simulink model "HQEV_MiL_20160830_integrate"  (Simulink 8.3)
settings: Solver=FixedStepDiscrete  StartTime=0.0  StopTime=inf  FixedStep=0.01  RelTol=1e-3
PostLoadFcn:
  | , if any(exist('dsrtsu_mdlpostloadfcn', 'file') == [2, 3, 6]), try dsrtsu_mdlpostloadfcn('Execute', bdroot); catch fprintf('Error in PostLoadFcn (dsrtsu_mdlpostloadfcn) for model "%s":\n %s\n', bdroot, lasterr); end, end,
values from neighbouring files (symbols this model uses):
  Bat_C_Ah = 36    [parameter_V1.mat]
  Bat_ocv_xIndex = [5 10 20 30 40 50 60 70 80 90 95]    [parameter_V1.mat]
  Bat_ocv_z = [329 332 340 345 347 351 358 372 377 386 391]    [parameter_V1.mat]
  Bat_R_ohm_z = [4.41 3.46 1.57 1.07 0.76 0.63 0.55 0.44 0.41 0.4 0.4 3.14 ... (66 elements, 11x6)]    [parameter_V1.mat]
  Bat_SOC_Init = 90    [parameter_V1.mat]
  Env_hum_pct_Ambient = 30    [parameter_V1.mat]
  Env_Slope_deg = 0    [parameter_V1.mat]
  Env_Temp_degC_Ambient = 25    [parameter_V1.mat]
  Env_v_kmph_HWind = 0    [parameter_V1.mat]
  Reducer_F_i = 7.23    [parameter_V1.mat]
  Reducer_R_i = 7.23    [parameter_V1.mat]
  Veh =     [parameter_V1.mat]
  Veh_A_m2_Fr = 2.246    [parameter_V1.mat]
  Veh_F_Brake =     [parameter_V1.mat]
  Veh_fac_AirDrag = 0.326    [parameter_V1.mat]
  Veh_fac_WhDragFrict_0 = 0.011    [parameter_V1.mat]
  Veh_g_mps2_C = 9.81    [parameter_V1.mat]
  Veh_GainBrake =     [parameter_V1.mat]
  Veh_h_m_COGHigh = 0.5    [parameter_V1.mat]
  Veh_J_kgm2_Wh = 1.3635    [parameter_V1.mat]
  Veh_L_m_AxlBas = 2.63    [parameter_V1.mat]
  Veh_M_kg = 1427    [parameter_V1.mat]
  Veh_mu_Brake = 0.4    [parameter_V1.mat]
  Veh_mu_Tyre =     [parameter_V1.mat]
  Veh_num_FrictPair = 8    [parameter_V1.mat]
  Veh_pct_Brk = 70    [parameter_V1.mat]
  Veh_r_dyn =     [parameter_V1.mat]
  Veh_r_m_BrkDisk = 0.136    [parameter_V1.mat]
  Veh_rho_kgpm3_Air = 1.2258    [parameter_V1.mat]
undefined symbols (not defined in the file or in its folder): DiscIntNeverNeededParam, p_bool_False_M, p_bool_True_M
libraries: BaseOperationLib_Browser x38, simulink x9, DTQC_lib x1, ERR_lib x1, MQM_lib x1, PTCL_lib x1, PUD_lib x1, TQD_lib x1, TQR_lib x1, VMM_lib x1, ACCA_lib x1, BBCA_lib x1
(part 4 of 15)

== system HQEV_MiL_20160830_integrate/MiL/Test_Integration/IC/IC ==
  In1 : Inport
  Bus Creator : BusCreator  Inputs=2
  Subsystem : Subsystem
  IC : Outport
  wires:
  In1/1 -> Subsystem/1(In1)
  Subsystem/1(HandBrakeSt) -> Bus Creator/1  "HandBrakeSt"
  Subsystem/2(DDSPS) -> Bus Creator/2  "DDSPS"
  Bus Creator/1 -> IC/1

== system HQEV_MiL_20160830_integrate/MiL/Test_Integration/MCU_FF/MCU ==
  In1 : Inport
  Bus Creator : BusCreator  Inputs=2
  MCU : Subsystem
  Signal : Subsystem
  Out1 : Outport
  wires:
  In1/1 -> Bus Creator/1, MCU/1(In1)
  MCU/1(out) -> Bus Creator/2
  Bus Creator/1 -> Signal/1(bus)
  Signal/1(Out1) -> Out1/1

== system HQEV_MiL_20160830_integrate/MiL/Test_Integration/MCU_RR/MCU ==
  In1 : Inport
  Bus Creator : BusCreator  Inputs=2
  MCU : Subsystem
  Signal : Subsystem
  Out1 : Outport
  wires:
  In1/1 -> Bus Creator/1, MCU/1(In1)
  MCU/1(Out1) -> Bus Creator/2
  Signal/1(Out1) -> Out1/1
  Bus Creator/1 -> Signal/1(in)

== system HQEV_MiL_20160830_integrate/MiL/Test_Integration/Motor_FF/Motor ==
  In1 : Inport
  Bus Creator : BusCreator  Inputs=6
  Bus Selector : BusSelector  OutputSignals=Reducer_F.FD1_spd_in,MCU_F.MCU1_trq_req,HCU.HCU_RapidDischargeCmdToMCU1,Battery.Battery_Voltage,BMS.BMS_MainPlusContactorCoilState,BMS.BMS_PrechargeContactorCoilState,BMS.BMS_MainMinusContactorCoilState,BMS.BMS_ChargePlusContactorCoilState,BMS.BMS_ChargeMinusContactorCoilState,Charger.Charger_Status
  Motor : Subsystem
  Out1 : Outport
  wires:
  In1/1 -> Bus Selector/1
  Motor/1(n_Motor) -> Bus Creator/1  "EM1_spd"
  Motor/2(P_Motor_elec) -> Bus Creator/2  "EM1_pwr_elec"
  Motor/3(T_out) -> Bus Creator/3  "EM1_trq_out"
  Motor/4(J_out) -> Bus Creator/4  "EM1_J_out"
  Motor/5(P_Motor_loss) -> Bus Creator/5  "EM1_pwr_loss"
  Motor/6(U_TMCap) -> Bus Creator/6  "EM1_U"
  Bus Creator/1 -> Out1/1
  Bus Selector/1 -> Motor/1(n_FD_in)  "<FD1_spd_in>"
  Bus Selector/2 -> Motor/2(T_req)  "<MCU1_trq_req>"
  Bus Selector/5 -> Motor/5(MainPos_Contactor)  "<BMS_MainPlusContactorCoilState>"
  Bus Selector/6 -> Motor/6(PreCharg_Contactor)  "<BMS_PrechargeContactorCoilState>"
  Bus Selector/7 -> Motor/7(MainNeg_Contactor)  "<BMS_MainMinusContactorCoilState>"
  Bus Selector/3 -> Motor/3(RapidDischargeEnable)  "<HCU_RapidDischargeCmdToMCU1>"
  Bus Selector/4 -> Motor/4(Battery_Voltage)  "<Battery_Voltage>"
  Bus Selector/8 -> Motor/8(BMS_ChargePlusContactorCoilState)  "<BMS_ChargePlusContactorCoilState>"
  Bus Selector/9 -> Motor/9(BMS_ChargeMinusContactorCoilState)  "<BMS_ChargeMinusContactorCoilState>"
  Bus Selector/10 -> Motor/10(Charger_Status)  "<Charger_Status>"

== system HQEV_MiL_20160830_integrate/MiL/Test_Integration/Motor_RR/Motor ==
  In1 : Inport
  Bus Creator : BusCreator  Inputs=6
  Bus Selector : BusSelector  OutputSignals=Reducer_R.FD2_spd_in,MCU_R.MCU2_trq_req,HCU.HCU_RapidDischargeCmdToMCU2,Battery.Battery_Voltage,BMS.BMS_MainPlusContactorCoilState,BMS.BMS_PrechargeContactorCoilState,BMS.BMS_MainMinusContactorCoilState,BMS.BMS_ChargePlusContactorCoilState,BMS.BMS_ChargeMinusContactorCoilState,Charger.Charger_Status
  Motor1 : Subsystem
  Out1 : Outport
  wires:
  In1/1 -> Bus Selector/1
  Motor1/1(n_Motor) -> Bus Creator/1  "EM2_spd"
  Motor1/2(P_Motor_elec) -> Bus Creator/2  "EM2_pwr_elec"
  Motor1/3(T_out) -> Bus Creator/3  "EM2_trq_out"
  Motor1/4(J_out) -> Bus Creator/4  "EM2_J_out"
  Motor1/5(P_Motor_loss) -> Bus Creator/5  "EM2_pwr_loss"
  Motor1/6(U_TMCap) -> Bus Creator/6  "EM2_U"
  Bus Creator/1 -> Out1/1
  Bus Selector/1 -> Motor1/1(n_FD_in)  "<FD2_spd_in>"
  Bus Selector/2 -> Motor1/2(T_req)  "<MCU2_trq_req>"
  Bus Selector/3 -> Motor1/3(RapidDischargeEnable)  "<HCU_RapidDischargeCmdToMCU2>"
  Bus Selector/4 -> Motor1/4(Battery_Voltage)  "<Battery_Voltage>"
  Bus Selector/5 -> Motor1/5(MainPos_Contactor)  "<BMS_MainPlusContactorCoilState>"
  Bus Selector/6 -> Motor1/6(PreCharg_Contactor)  "<BMS_PrechargeContactorCoilState>"
  Bus Selector/7 -> Motor1/7(MainNeg_Contactor)  "<BMS_MainMinusContactorCoilState>"
  Bus Selector/8 -> Motor1/8(BMS_ChargePlusContactorCoilState)  "<BMS_ChargePlusContactorCoilState>"
  Bus Selector/9 -> Motor1/9(BMS_ChargeMinusContactorCoilState)  "<BMS_ChargeMinusContactorCoilState>"
  Bus Selector/10 -> Motor1/10(Charger_Status)  "<Charger_Status>"

== system HQEV_MiL_20160830_integrate/MiL/Test_Integration/Reducer_F/FinalDrive ==
  In1 : Inport
  Bus Creator : BusCreator  Inputs=3
  Bus Selector1 : BusSelector  OutputSignals=Motor_F.EM1_trq_out,Vehicle.n_Wh,Motor_F.EM1_J_out
  FinalDrive : Subsystem
  Out : Outport
  wires:
  FinalDrive/1("T_out ") -> Bus Creator/1  "FD1_trq_out"
  FinalDrive/2(n_in) -> Bus Creator/2  "FD1_spd_in"
  FinalDrive/3("J_out ") -> Bus Creator/3  "FD1_J_out"
  Bus Creator/1 -> Out/1
  In1/1 -> Bus Selector1/1
  Bus Selector1/1 -> FinalDrive/1(T_in)  "<EM1_trq_out>"
  Bus Selector1/2 -> FinalDrive/2(n_Wheel)  "<n_Wh>"
  Bus Selector1/3 -> FinalDrive/3(J_in)  "<EM1_J_out>"

== system HQEV_MiL_20160830_integrate/MiL/Test_Integration/Reducer_R/FinalDrive ==
  In1 : Inport
  Bus Creator : BusCreator  Inputs=3
  Bus Selector1 : BusSelector  OutputSignals=Motor_R.EM2_trq_out,Vehicle.n_Wh,Motor_R.EM2_J_out
  FinalDrive : Subsystem
  Out : Outport
  wires:
  Bus Selector1/3 -> FinalDrive/3(J_in [kg*m^2])  "<EM2_J_out>"
  Bus Selector1/2 -> FinalDrive/2(n_Wheel)  "<n_Wh>"
  Bus Selector1/1 -> FinalDrive/1(T_in)  "<EM2_trq_out>"
  In1/1 -> Bus Selector1/1
  Bus Creator/1 -> Out/1
  FinalDrive/3(J_out [kg*m^2]) -> Bus Creator/3  "FD2_J_out"
  FinalDrive/2(n_in) -> Bus Creator/2  "FD2_spd_in"
  FinalDrive/1(T_out [Nm]) -> Bus Creator/1  "FD2_trq_out"

== system HQEV_MiL_20160830_integrate/MiL/Test_Integration/Thermal/Thermal ==
  In1 : Inport
  Bus Creator : BusCreator  Inputs=5
  Bus Selector : BusSelector  OutputSignals=HCU.EM1PumpCmd_pct,HCU.EM2PumpCmd_pct,Motor_F.EM1_pwr_loss,Motor_R.EM2_pwr_loss,HCU.LowSpdFanCmd_na,HCU.HighSpdFanCmd_na,Charger.Charger_pwr_out,DCDC.DCDC_pwr_Loss,HCU.BatPumpCmd_pct,HCU.HCU_BatteryPackCoolRequest,HCU.PTC_PWM_pct,Battery.Battery_Power_loss,IO.BatTempIndex
  Subsystem : Subsystem
  Out1 : Outport
  wires:
  Bus Creator/1 -> Out1/1
  Subsystem/1(Motor_F_Temp) -> Bus Creator/1  "Motor_F_Temp"
  Subsystem/2(Motor_R_Temp) -> Bus Creator/2  "Motor_R_Temp"
  Subsystem/3(DCDC_Temp) -> Bus Creator/3  "DCDC_Temp"
  Subsystem/4(Charger_Temp) -> Bus Creator/4  "Charger_Temp"
  Subsystem/5(Battery_Temp) -> Bus Creator/5  "Battery_Temp"
  In1/1 -> Bus Selector/1
  Bus Selector/1 -> Subsystem/1(PWM_Pump1)  "<EM1PumpCmd_pct>"
  Bus Selector/2 -> Subsystem/2(PWM_Pump2)  "<EM2PumpCmd_pct>"
  Bus Selector/3 -> Subsystem/3(pwr_Motor1Loss)  "<EM1_pwr_loss>"
  Bus Selector/4 -> Subsystem/4(pwr_Motor2Loss)  "<EM2_pwr_loss>"
  Bus Selector/5 -> Subsystem/5(LowSpdFan_na)  "<LowSpdFanCmd_na>"
  Bus Selector/6 -> Subsystem/6(HighSpdFan_na)  "<HighSpdFanCmd_na>"
  Bus Selector/7 -> Subsystem/7(pwr_ChargerLoss)  "<Charger_pwr_out>"
  Bus Selector/8 -> Subsystem/8(pwr_DCDCLoss)  "<DCDC_pwr_Loss>"
  Bus Selector/9 -> Subsystem/9(PWM_BatteryPump)  "<BatPumpCmd_pct>"
  Bus Selector/10 -> Subsystem/10(AC_OnOff)  "<HCU_BatteryPackCoolRequest>"
  Bus Selector/11 -> Subsystem/11(PWM_PTC)  "<PTC_PWM_pct>"
  Bus Selector/12 -> Subsystem/12(pwr_BatteryLoss)  "<Battery_Power_loss>"
  Bus Selector/13 -> Subsystem/13(BatTempIndex)  "<BatTempIndex>"

== system HQEV_MiL_20160830_integrate/MiL/Test_Integration/Vehicle/Vehicle ==
  In1 : Inport
  Add : Sum
  Bus Creator : BusCreator
  Bus Selector : BusSelector  OutputSignals=Reducer_F.FD1_trq_out,Reducer_R.FD2_trq_out,Drv.signal1.BrkPed_pct,Env.v_Hwind,Reducer_F.FD1_J_out,Reducer_R.FD2_J_out
  Constant1 : Constant  Value=0
  Constant3 : Constant  Value=0
  Vehicle : Subsystem
  Out2 : Outport
  wires:
  Vehicle/1(n_Wh) -> Bus Creator/1  "n_Wh"
  Vehicle/2(dist [km]) -> Bus Creator/2  "dist"
  Vehicle/3(v_Veh [km/h]) -> Bus Creator/3  "v_Veh"
  Constant3/1 -> Vehicle/6(m_add)
  Bus Creator/1 -> Out2/1  "Vehicle"
  Vehicle/4(acc) -> Bus Creator/4  "acc"
  In1/1 -> Bus Selector/1
  Bus Selector/1 -> Vehicle/1("T_inFront ")  "<FD1_trq_out>"
  Bus Selector/2 -> Vehicle/2("T_inRear ")  "<FD2_trq_out>"
  Bus Selector/3 -> Vehicle/3(Sig_Brake)  "<BrkPed_pct>"
  Bus Selector/4 -> Vehicle/4(v_Hwind_mps)  "<v_Hwind>"
  Bus Selector/5 -> Add/1  "<FD1_J_out>"
  Bus Selector/6 -> Add/2  "<FD2_J_out>"
  Add/1 -> Vehicle/5(J_in)
  Constant1/1 -> Vehicle/7(Slope_deg)

== system HQEV_MiL_20160830_integrate/MiL/Test_Integration/AC/AirConditioning/ACIndication ==
  Constant8 : Constant  Value=0
  out : Outport
  wires:
  Constant8/1 -> out/1

== system HQEV_MiL_20160830_integrate/MiL/Test_Integration/AC/AirConditioning/AC_CompressorOnRequest ==
  Constant : Constant  Value=0
  out : Outport
  wires:
  Constant/1 -> out/1

== system HQEV_MiL_20160830_integrate/MiL/Test_Integration/AC/AirConditioning/AC_FanRequest ==
  Constant6 : Constant  Value=0
  out : Outport
  wires:
  Constant6/1 -> out/1

== system HQEV_MiL_20160830_integrate/MiL/Test_Integration/AC/AirConditioning/AC_PTCStatus ==
  Constant6 : Constant  Value=0
  out : Outport
  wires:
  Constant6/1 -> out/1

== system HQEV_MiL_20160830_integrate/MiL/Test_Integration/AC/AirConditioning/AC_PowerConsumptionH ==
  Constant10 : Constant
  out : Outport
  wires:
  Constant10/1 -> out/1

== system HQEV_MiL_20160830_integrate/MiL/Test_Integration/AC/AirConditioning/AC_PowerConsumptionL ==
  Constant2 : Constant  Value=0
  out : Outport
  wires:
  Constant2/1 -> out/1

== system HQEV_MiL_20160830_integrate/MiL/Test_Integration/AC/AirConditioning/AC_ShutdownEnableH ==
  Constant3 : Constant
  out : Outport
  wires:
  Constant3/1 -> out/1

== system HQEV_MiL_20160830_integrate/MiL/Test_Integration/AC/AirConditioning/AC_Status ==
  Constant1 : Constant  Value=0
  out : Outport
  wires:
  Constant1/1 -> out/1

== system HQEV_MiL_20160830_integrate/MiL/Test_Integration/AC/AirConditioning/AC_shutdownEnableL ==
  Constant3 : Constant
  out : Outport
  wires:
  Constant3/1 -> out/1

== system HQEV_MiL_20160830_integrate/MiL/Test_Integration/AC/AirConditioning/BLWLevelIndication ==
  Constant9 : Constant  Value=0
  out : Outport
  wires:
  Constant9/1 -> out/1

== system HQEV_MiL_20160830_integrate/MiL/Test_Integration/AC/AirConditioning/Checksum_AC_1 ==
  Constant : Constant  Value=0
  out : Outport
  wires:
  Constant/1 -> out/1

== system HQEV_MiL_20160830_integrate/MiL/Test_Integration/AC/AirConditioning/LiveCounter_AC_1 ==
  Constant : Constant  Value=0
  out : Outport
  wires:
  Constant/1 -> out/1

== system HQEV_MiL_20160830_integrate/MiL/Test_Integration/AC/AirConditioning/OutsideTemperatureIndication ==
  Constant10 : Constant  Value=25
  out : Outport
  wires:
  Constant10/1 -> out/1

== system HQEV_MiL_20160830_integrate/MiL/Test_Integration/ACC/ACC/Output ==
  HCU_ActualMotoringTorque : Inport
  HCU_MaxAvaiblleMotoringTorque : Inport  Port=2
  HCUStatus : Inport  Port=3
  AccelerationPedalPosition : Inport  Port=4
  CalculatedAccelerationPedalPosition : Inport  Port=5
  KickdownRequest : Inport  Port=6
  BrakeSwitch : Inport  Port=7
  AccelerationPedalOverride : Inport  Port=8
  CCMainSwitch : Inport  Port=9
  CCCancelSwitch : Inport  Port=10
  CCSetOrCoastSwitch : Inport  Port=11
  CCResumeOrAccelerateSwitch : Inport  Port=12
  HCUResponseACC : Inport  Port=13
  HeadwaySwitch : Inport  Port=14
  CCSwitchError : Inport  Port=15
  LeverInfo : Inport  Port=16
  IO_Input : Inport  Port=17
  Bus Selector : BusSelector  OutputSignals=IO.ACC_ErrorStatus,IO.ACC_Status,IO.ACC_TorqueRequest,IO.ACC_StatusTorqueRequest,IO.ACC_StatusACCDecelerationRequest
  Constant4 : Constant  Value=0
  Terminator{,1..15} (16 alike) : Terminator
  ACC_ErrorStatus : Outport
  ACC_Status : Outport  Port=2
  ACC_TorqueRequest : Outport  Port=3
  ACC_StatusTorqueRequest : Outport  Port=4
  ACC_DecelerationRequest : Outport  Port=5
  ACC_StatusACCDecelerationRequest : Outport  Port=6
  wires:
  HCU_ActualMotoringTorque/1 -> Terminator/1
  HCU_MaxAvaiblleMotoringTorque/1 -> Terminator1/1
  HCUStatus/1 -> Terminator2/1
  AccelerationPedalPosition/1 -> Terminator3/1
  CalculatedAccelerationPedalPosition/1 -> Terminator4/1
  KickdownRequest/1 -> Terminator5/1
  BrakeSwitch/1 -> Terminator6/1
  AccelerationPedalOverride/1 -> Terminator7/1
  CCMainSwitch/1 -> Terminator8/1
  CCCancelSwitch/1 -> Terminator9/1
  CCSetOrCoastSwitch/1 -> Terminator10/1
  CCResumeOrAccelerateSwitch/1 -> Terminator11/1
  HCUResponseACC/1 -> Terminator12/1
  HeadwaySwitch/1 -> Terminator13/1
  CCSwitchError/1 -> Terminator14/1
  LeverInfo/1 -> Terminator15/1
  IO_Input/1 -> Bus Selector/1
  Constant4/1 -> ACC_DecelerationRequest/1
  Bus Selector/1 -> ACC_ErrorStatus/1  "<ACC_ErrorStatus>"
  Bus Selector/2 -> ACC_Status/1  "<ACC_Status>"
  Bus Selector/3 -> ACC_TorqueRequest/1  "<ACC_TorqueRequest>"
  Bus Selector/4 -> ACC_StatusTorqueRequest/1  "<ACC_StatusTorqueRequest>"
  Bus Selector/5 -> ACC_StatusACCDecelerationRequest/1  "<ACC_StatusACCDecelerationRequest>"

== system HQEV_MiL_20160830_integrate/MiL/Test_Integration/Accessory/Accessory/Subsystem ==
  In1 : Inport
  vacuum booster : Subsystem
  vacuum degree : Outport
  wires:
  vacuum booster/1(vacuum degree) -> vacuum degree/1
  In1/1 -> vacuum booster/1(In1)

== system HQEV_MiL_20160830_integrate/MiL/Test_Integration/BCM/BCM/Check ==
  In1 : Inport
  Subsystem : Subsystem
  Subsystem1 : Subsystem
  Subsystem2 : Subsystem
  Subsystem3 : Subsystem
  Subsystem4 : Subsystem
  Subsystem5 : Subsystem
  Subsystem6 : Subsystem
  Terminator : Terminator
  BCM_HighBeamCmd : Outport
  DriverDoorSt : Outport  Port=2
  WiperStatus : Outport  Port=3
  Checksum_PSC : Outport  Port=4
  DataBytes : Outport  Port=5
  LiveCounter_PSC : Outport  Port=6
  MessageType : Outport  Port=7
  wires:
  In1/1 -> Terminator/1
  Subsystem/1(Checksum_PSC) -> Checksum_PSC/1
  Subsystem1/1(DataBytes) -> DataBytes/1
  Subsystem2/1(LiveCounter_PSC) -> LiveCounter_PSC/1
  Subsystem3/1(MessageType) -> MessageType/1
  Subsystem4/1(BCM_HighBeamCmd) -> BCM_HighBeamCmd/1
  Subsystem5/1(DriverDoorSt) -> DriverDoorSt/1
  Subsystem6/1(WiperStatus) -> WiperStatus/1

== system HQEV_MiL_20160830_integrate/MiL/Test_Integration/BMS/BMS/BMS ==
  In1 : Inport
  BMS : Subsystem
  Bus Creator : BusCreator  Inputs=27
  Bus Selector : BusSelector  OutputSignals=HCU.HCU_MainPosContactorControl,HCU.HCU_MainNegContactorControl,HCU.HCU_PrechargeContactorControl,HCU.HCU_ChargePosContactorControl,HCU.HCU_ChargeNegContactorControl,HCU.HCU_ChargeConnectStatus,Battery.SOC,Battery.Battery_Temp,HCU.HCU_ChargePermission,HCU.HCU_ChargeHeatingPermission,Battery.SOH,Thermal.Battery_Temp,IO.BMS_InsulationMonitorWarning
  Compare To Constant : simulink/Logic and Bit Operations/Compare To Constant  SystemSampleTime=-1  relop===  const=2  LogicOutDataTypeMode=boolean
  Compare To Constant1 : simulink/Logic and Bit Operations/Compare To Constant  SystemSampleTime=-1  relop===  const=1  LogicOutDataTypeMode=boolean
  Out : Outport
  wires:
  Bus Creator/1 -> Out/1
  BMS/1(MainPosContactorState) -> Bus Creator/1  "MainPlusContactorState"
  BMS/2(MainNegContactorCoilState) -> Bus Creator/2  "MainMinusContactorCoilState"
  BMS/3(PrechargeContactorCoilState) -> Bus Creator/3  "PrechargeContactorCoilState"
  BMS/4(ChargPosContactorState) -> Bus Creator/4  "ChargePlusContactorState"
  BMS/5(ChargNegContactorCoilState) -> Bus Creator/5  "ChargeMinusContactorCoilState"
  BMS/6(BMS_ChargeRequest) -> Bus Creator/6  "BMS_ChargeRequest"
  BMS/7(BMS_ChargeStationOutputCurrent) -> Bus Creator/7  "BMS_ChargeStationOutputCurrent"
  BMS/8(BMS_ChargeStationOutputVoltage) -> Bus Creator/8  "BMS_ChargeStationOutputVoltage"
  BMS/9(BMS_InstantPowerConsumption) -> Bus Creator/9  "BMS_InstantPowerConsumption"
  BMS/10(BMS_ChargeStationParameterConfigStatus) -> Bus Creator/10  "BMS_ChargeStationParameterConfigStatus"
  BMS/11(BMS_ChargeStationStatus) -> Bus Creator/11  "BMS_ChargeStationStatus"
  BMS/12(BMS_RemainingChargeTime) -> Bus Creator/12  "BMS_RemainingChargeTime"
  BMS/13(BMS_InsulationMonitorWarning) -> Bus Creator/13  "BMS_InsulationMonitorWarning"
  BMS/14(BMS_ChargeStationHandShakeStatus) -> Bus Creator/14  "BMS_ChargeStationHandShakeStatus"
  BMS/15(BatteryChargePowerAvailable_10) -> Bus Creator/15  "BatteryChargePowerAvailable_10"
  BMS/16(BMS_BatteryDischargePowerAvailable_10) -> Bus Creator/16  "BMS_BatteryDischargePowerAvailable_10"
  BMS/17(BMS_BatteryChargePowerAvailable_2) -> Bus Creator/17  "BMS_BatteryChargePowerAvailable_2"
  BMS/18(BMS_BatteryDischargePowerAvailable_2) -> Bus Creator/18  "BMS_BatteryDischargePowerAvailable_2"
  BMS/19(BMS_SOH) -> Bus Creator/19  "BMS_SOH"
  BMS/20(BMS_SOC) -> Bus Creator/20  "BMS_SOC"
  BMS/21(BMS RemainingEnergyRatio) -> Bus Creator/21  "BMS RemainingEnergyRatio"
  BMS/22(Bat_temp_Max) -> Bus Creator/22  "Bat_temp_Max"
  BMS/23(Bat_temp_Min) -> Bus Creator/23  "Bat_temp_Min"
  BMS/24(Bat_temp_ave) -> Bus Creator/24  "Bat_temp_ave"
  BMS/25(Bat_temp_water) -> Bus Creator/25  "Bat_temp_water"
  BMS/26(BMS_HeatingRequest) -> Bus Creator/26  "BMS_HeatingRequest"
  In1/1 -> Bus Selector/1
  Bus Selector/1 -> BMS/1(MainPosContactorCtrl)  "<HCU_MainPosContactorControl>"
  Bus Selector/2 -> BMS/2(MainNegContactorCtrl)  "<HCU_MainNegContactorControl>"
  Bus Selector/3 -> BMS/3(PrechargContactorCtrl)  "<HCU_PrechargeContactorControl>"
  Bus Selector/4 -> BMS/4(ChargPosContactorCtrl)  "<HCU_ChargePosContactorControl>"
  Bus Selector/5 -> BMS/5(ChargeNegContactorCtrl)  "<HCU_ChargeNegContactorControl>"
  Bus Selector/7 -> BMS/8(SOC)  "<SOC>"
  Bus Selector/8 -> BMS/9(Bat_temp)  "<Battery_Temp>"
  Bus Selector/9 -> BMS/10(HCU_ChargePermission)  "<HCU_ChargePermission>"
  Bus Selector/11 -> BMS/12(SOH)  "<SOH>"
  BMS/27(BMS_ChargeStatus) -> Bus Creator/27  "BMS_ChargeStatus"
  Bus Selector/6 -> Compare To Constant1/1, Compare To Constant/1  "<HCU_ChargeConnectStatus>"
  Compare To Constant/1 -> BMS/6(CC)
  Compare To Constant1/1 -> BMS/7(CC2)
  Bus Selector/12 -> BMS/13(Battery_Temp)  "<Battery_Temp>"
  Bus Selector/10 -> BMS/11(HCU_ChargeHeatingPermission)  "<HCU_ChargeHeatingPermission>"
  Bus Selector/13 -> BMS/14(BMS_InsulationMonitorWarningIN)  "<BMS_InsulationMonitorWarning>"

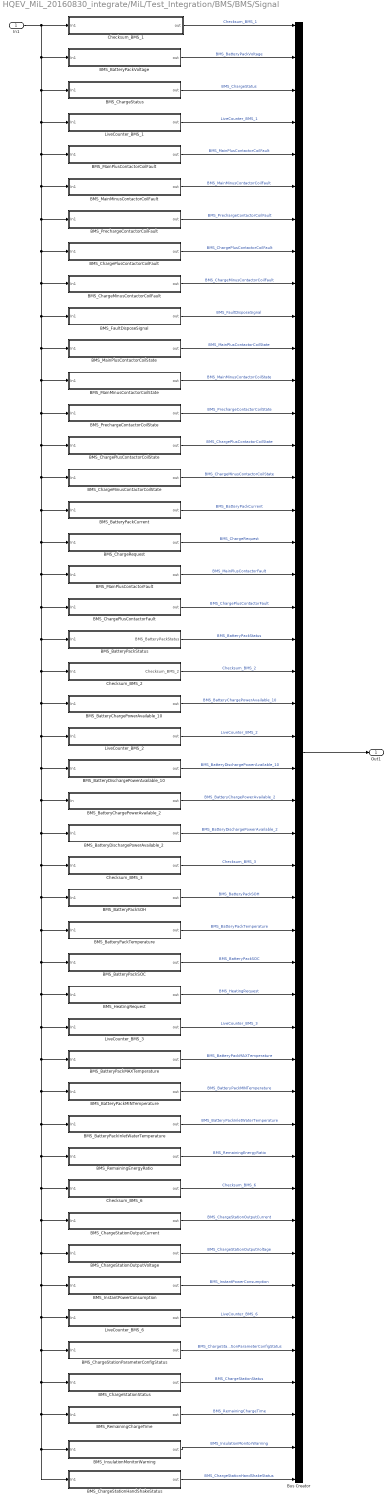
== system HQEV_MiL_20160830_integrate/MiL/Test_Integration/BMS/BMS/Signal ==
  In1 : Inport
  BMS_BatteryChargePowerAvailable_10 : Subsystem
  BMS_BatteryChargePowerAvailable_2 : Subsystem
  BMS_BatteryDischargePowerAvailable_10 : Subsystem
  BMS_BatteryDischargePowerAvailable_2 : Subsystem
  BMS_BatteryPackCurrent : Subsystem
  BMS_BatteryPackInletWaterTemperature : Subsystem
  BMS_BatteryPackMAXTemperature : Subsystem
  BMS_BatteryPackMINTemperature : Subsystem
  BMS_BatteryPackSOC : Subsystem
  BMS_BatteryPackSOH : Subsystem
  BMS_BatteryPackStatus : Subsystem
  BMS_BatteryPackTemperature : Subsystem
  BMS_BatteryPackVoltage : Subsystem
  BMS_ChargeMinusContactorCoilFault : Subsystem
  BMS_ChargeMinusContactorCoilState : Subsystem
  BMS_ChargePlusContactorCoilFault : Subsystem
  BMS_ChargePlusContactorCoilState : Subsystem
  BMS_ChargePlusContactorFault : Subsystem
  BMS_ChargeRequest : Subsystem
  BMS_ChargeStationHandShakeStatus : Subsystem
  BMS_ChargeStationOutputCurrent : Subsystem
  BMS_ChargeStationOutputVoltage : Subsystem
  BMS_ChargeStationParameterConfigStatus : Subsystem
  BMS_ChargeStationStatus : Subsystem
  BMS_ChargeStatus : Subsystem
  BMS_FaultDisposeSignal : Subsystem
  BMS_HeatingRequest : Subsystem
  BMS_InstantPowerConsumption : Subsystem
  BMS_InsulationMonitorWarning : Subsystem
  BMS_MainMinusContactorCoilFault : Subsystem
  BMS_MainMinusContactorCoilState : Subsystem
  BMS_MainPlusContactorCoilFault : Subsystem
  BMS_MainPlusContactorCoilState : Subsystem
  BMS_MainPlusContactorFault : Subsystem
  BMS_PrechargeContactorCoilFault : Subsystem
  BMS_PrechargeContactorCoilState : Subsystem
  BMS_RemainingChargeTime : Subsystem
  BMS_RemainingEnergyRatio : Subsystem
  Bus Creator : BusCreator  Inputs=46
  Checksum_BMS_1 : Subsystem
  Checksum_BMS_2 : Subsystem
  Checksum_BMS_3 : Subsystem
  Checksum_BMS_6 : Subsystem
  LiveCounter_BMS_1 : Subsystem
  LiveCounter_BMS_2 : Subsystem
  LiveCounter_BMS_3 : Subsystem
  LiveCounter_BMS_6 : Subsystem
  Out1 : Outport
  wires:
  Checksum_BMS_1/1(out) -> Bus Creator/1  "Checksum_BMS_1"
  BMS_BatteryPackVoltage/1(out) -> Bus Creator/2  "BMS_BatteryPackVoltage"
  BMS_ChargeStatus/1(out) -> Bus Creator/3  "BMS_ChargeStatus"
  LiveCounter_BMS_1/1(out) -> Bus Creator/4  "LiveCounter_BMS_1"
  BMS_ChargeStationHandShakeStatus/1(out) -> Bus Creator/46  "BMS_ChargeStationHandShakeStatus"
  BMS_InsulationMonitorWarning/1(out) -> Bus Creator/45  "BMS_InsulationMonitorWarning"
  BMS_RemainingChargeTime/1(out) -> Bus Creator/44  "BMS_RemainingChargeTime"
  BMS_ChargeStationStatus/1(out) -> Bus Creator/43  "BMS_ChargeStationStatus"
  BMS_ChargeStationParameterConfigStatus/1(out) -> Bus Creator/42  "BMS_ChargeStationParameterConfigStatus"
  LiveCounter_BMS_6/1(out) -> Bus Creator/41  "LiveCounter_BMS_6"
  BMS_InstantPowerConsumption/1(out) -> Bus Creator/40  "BMS_InstantPowerConsumption"
  BMS_ChargeStationOutputVoltage/1(out) -> Bus Creator/39  "BMS_ChargeStationOutputVoltage"
  BMS_ChargeStationOutputCurrent/1(out) -> Bus Creator/38  "BMS_ChargeStationOutputCurrent"
  Checksum_BMS_6/1(out) -> Bus Creator/37  "Checksum_BMS_6"
  BMS_RemainingEnergyRatio/1(out) -> Bus Creator/36  "BMS_RemainingEnergyRatio"
  BMS_BatteryPackInletWaterTemperature/1(out) -> Bus Creator/35  "BMS_BatteryPackInletWaterTemperature"
  BMS_BatteryPackMINTemperature/1(out) -> Bus Creator/34  "BMS_BatteryPackMINTemperature"
  BMS_BatteryPackMAXTemperature/1(out) -> Bus Creator/33  "BMS_BatteryPackMAXTemperature"
  LiveCounter_BMS_3/1(out) -> Bus Creator/32  "LiveCounter_BMS_3"
  BMS_HeatingRequest/1(out) -> Bus Creator/31  "BMS_HeatingRequest"
  BMS_BatteryPackSOC/1(out) -> Bus Creator/30  "BMS_BatteryPackSOC"
  BMS_BatteryPackTemperature/1(out) -> Bus Creator/29  "BMS_BatteryPackTemperature"
  BMS_BatteryPackSOH/1(out) -> Bus Creator/28  "BMS_BatteryPackSOH"
  Checksum_BMS_3/1(out) -> Bus Creator/27  "Checksum_BMS_3"
  BMS_BatteryDischargePowerAvailable_2/1(out) -> Bus Creator/26  "BMS_BatteryDischargePowerAvailable_2"
  BMS_BatteryChargePowerAvailable_2/1(out) -> Bus Creator/25  "BMS_BatteryChargePowerAvailable_2"
  BMS_BatteryDischargePowerAvailable_10/1(out) -> Bus Creator/24  "BMS_BatteryDischargePowerAvailable_10"
  LiveCounter_BMS_2/1(out) -> Bus Creator/23  "LiveCounter_BMS_2"
  BMS_BatteryChargePowerAvailable_10/1(out) -> Bus Creator/22  "BMS_BatteryChargePowerAvailable_10"
  Checksum_BMS_2/1(Checksum_BMS_2) -> Bus Creator/21  "Checksum_BMS_2"
  BMS_BatteryPackStatus/1(BMS_BatteryPackStatus) -> Bus Creator/20  "BMS_BatteryPackStatus"
  BMS_ChargePlusContactorFault/1(out) -> Bus Creator/19  "BMS_ChargePlusContactorFault"
  BMS_MainPlusContactorFault/1(out) -> Bus Creator/18  "BMS_MainPlusContactorFault"
  BMS_ChargeRequest/1(out) -> Bus Creator/17  "BMS_ChargeRequest"
  BMS_BatteryPackCurrent/1(out) -> Bus Creator/16  "BMS_BatteryPackCurrent"
  BMS_ChargeMinusContactorCoilState/1(out) -> Bus Creator/15  "BMS_ChargeMinusContactorCoilState"
  BMS_ChargePlusContactorCoilState/1(out) -> Bus Creator/14  "BMS_ChargePlusContactorCoilState"
  BMS_PrechargeContactorCoilState/1(out) -> Bus Creator/13  "BMS_PrechargeContactorCoilState"
  BMS_MainMinusContactorCoilState/1(out) -> Bus Creator/12  "BMS_MainMinusContactorCoilState"
  BMS_MainPlusContactorCoilState/1(out) -> Bus Creator/11  "BMS_MainPlusContactorCoilState"
  BMS_FaultDisposeSignal/1(out) -> Bus Creator/10  "BMS_FaultDisposeSignal"
  BMS_ChargeMinusContactorCoilFault/1(out) -> Bus Creator/9  "BMS_ChargeMinusContactorCoilFault"
  BMS_ChargePlusContactorCoilFault/1(out) -> Bus Creator/8  "BMS_ChargePlusContactorCoilFault"
  BMS_PrechargeContactorCoilFault/1(out) -> Bus Creator/7  "BMS_PrechargeContactorCoilFault"
  BMS_MainMinusContactorCoilFault/1(out) -> Bus Creator/6  "BMS_MainMinusContactorCoilFault"
  BMS_MainPlusContactorCoilFault/1(out) -> Bus Creator/5  "BMS_MainPlusContactorCoilFault"
  In1/1 -> Checksum_BMS_1/1(In1), BMS_BatteryPackVoltage/1(In1), BMS_ChargeStatus/1(In1), LiveCounter_BMS_1/1(In1), BMS_MainPlusContactorCoilFault/1(In1), BMS_MainMinusContactorCoilFault/1(In1), BMS_PrechargeContactorCoilFault/1(In1), BMS_ChargePlusContactorCoilFault/1(In1), BMS_ChargeMinusContactorCoilFault/1(In1), BMS_FaultDisposeSignal/1(In1), BMS_MainPlusContactorCoilState/1(In1), BMS_MainMinusContactorCoilState/1(In1), BMS_PrechargeContactorCoilState/1(In1), BMS_ChargePlusContactorCoilState/1(In1), BMS_ChargeMinusContactorCoilState/1(In1), BMS_BatteryPackCurrent/1(In1), BMS_ChargeRequest/1(In1), BMS_MainPlusContactorFault/1(In1), BMS_ChargePlusContactorFault/1(In1), BMS_BatteryPackStatus/1(In1), Checksum_BMS_2/1(In1), BMS_BatteryChargePowerAvailable_10/1(In1), LiveCounter_BMS_2/1(In1), BMS_BatteryDischargePowerAvailable_10/1(In1), BMS_BatteryChargePowerAvailable_2/1(In), BMS_BatteryDischargePowerAvailable_2/1(In1), Checksum_BMS_3/1(In1), BMS_BatteryPackSOH/1(In1), BMS_BatteryPackTemperature/1(In1), BMS_BatteryPackSOC/1(In1), BMS_HeatingRequest/1(In1), LiveCounter_BMS_3/1(In1), BMS_BatteryPackMAXTemperature/1(In1), BMS_BatteryPackMINTemperature/1(In1), BMS_BatteryPackInletWaterTemperature/1(In1), BMS_RemainingEnergyRatio/1(In1), Checksum_BMS_6/1(In1), BMS_ChargeStationOutputCurrent/1(In1), BMS_ChargeStationOutputVoltage/1(In1), BMS_InstantPowerConsumption/1(In1), LiveCounter_BMS_6/1(In1), BMS_ChargeStationParameterConfigStatus/1(In1), BMS_ChargeStationStatus/1(In1), BMS_RemainingChargeTime/1(In1), BMS_InsulationMonitorWarning/1(In1), BMS_ChargeStationHandShakeStatus/1(In1)
  Bus Creator/1 -> Out1/1

== system HQEV_MiL_20160830_integrate/MiL/Test_Integration/Battery/Battery/Battery ==
  EM1_pwr_elec : Inport
  EM2_pwr_elec : Inport  Port=2
  DCDC_pwr_in : Inport  Port=3
  AC_pwr_elec : Inport  Port=4
  Battery_Temp : Inport  Port=5
  SOCIndex : Inport  Port=6
  Charger_OutputVoltage : Inport  Port=7
  Charger_OutputCurrent : Inport  Port=8
  HCU_ChargerPermission : Inport  Port=9
  Battery_Output : Subsystem
  Constant : Constant  Value=100
  Constant1 : Constant  Value=30
  SOC_Subsystem : Subsystem
  Subsystem : Subsystem
  Battery_Voltage : Outport
  Battery_Current : Outport  Port=2
  SOC : Outport  Port=3
  SOH : Outport  Port=4
  Battery_Temperature : Outport  Port=5
  Battery_Power_loss : Outport  Port=6
  wires:
  Battery_Output/1(Battery_Voltage) -> Battery_Voltage/1
  Subsystem/1(Bat_pwr_out) -> Battery_Output/1(Bat_pwr_out)
  Battery_Output/3(Battery_Current) -> SOC_Subsystem/1(Battery_Current), Battery_Current/1
  Constant/1 -> SOH/1
  Constant1/1 -> Battery_Temperature/1
  Battery_Temp/1 -> Battery_Output/2(Battery_Temp)
  Battery_Output/2(Battery_Power_loss) -> Battery_Power_loss/1
  SOC_Subsystem/1(SOC) -> Battery_Output/3(SOC), SOC/1
  DCDC_pwr_in/1 -> Subsystem/3(DCDC_pwr_in)
  EM1_pwr_elec/1 -> Subsystem/1(EM1_pwr_elec)
  EM2_pwr_elec/1 -> Subsystem/2(EM2_pwr_elec)
  AC_pwr_elec/1 -> Subsystem/4(AC_pwr_elec)
  SOCIndex/1 -> SOC_Subsystem/2(SOCIndex)
  Charger_OutputVoltage/1 -> Subsystem/5(Charger_OutputVoltage)
  Charger_OutputCurrent/1 -> Subsystem/6(Charger_OutputCurrent)
  HCU_ChargerPermission/1 -> Subsystem/7(HCU_ChargerPermission)

== system HQEV_MiL_20160830_integrate/MiL/Test_Integration/Charger/Charger/Charger ==
  In : Inport
  Bus Creator : BusCreator  Inputs=6
  Bus Selector : BusSelector  OutputSignals=HCU.HCU_ChargeConnectStatus,HCU.HCU_ChargePermission,BMS.BMS_MainPlusContactorCoilState,HCU.HCU_ChargeHeatingPermission,BMS.BMS_MainMinusContactorCoilState,BMS.BMS_PrechargeContactorCoilState,BMS.BMS_ChargePlusContactorCoilState,BMS.BMS_ChargeMinusContactorCoilState
  Charger : Subsystem
  Constant1 : Constant  Value=2
  Constant3 : Constant  Value=220
  Product : Product  RndMeth=Zero
  Relational Operator : RelationalOperator  Operator===  OutDataTypeStr=boolean
  Out : Outport
  wires:
  Bus Creator/1 -> Out/1
  In/1 -> Charger/10(IO_In), Bus Selector/1
  Constant3/1 -> Charger/1(ACChargeStation_U)
  Bus Selector/8 -> Charger/9(BMS_ChargeNegContactorState)  "<BMS_ChargeMinusContactorCoilState>"
  Bus Selector/7 -> Charger/8(BMS_ChargePosContactorState)  "<BMS_ChargePlusContactorCoilState>"
  Bus Selector/6 -> Charger/7(BMS_PreChargeContactorState)  "<BMS_PrechargeContactorCoilState>"
  Bus Selector/5 -> Charger/6(BMS_MainNegContactorState)  "<BMS_MainMinusContactorCoilState>"
  Bus Selector/2 -> Charger/3(HCU_ChargePermission)  "<HCU_ChargePermission>"
  Charger/1(ChargerOutputVoltage) -> Bus Creator/1, Product/2  "Charger_OutputVoltage"
  Charger/2(ChargerStatus) -> Bus Creator/2  "Charger_Status"
  Charger/3(RechargeRequest) -> Bus Creator/3  "Charger_RechargeRequest"
  Charger/4(ChargerOutputCurrent) -> Bus Creator/4, Product/1  "Charger_OutputCurrent"
  Charger/5(ChargerTemperature) -> Bus Creator/5  "Charger_Temperature"
  Bus Selector/1 -> Relational Operator/1  "<HCU_ChargeConnectStatus>"
  Constant1/1 -> Relational Operator/2
  Relational Operator/1 -> Charger/2(CC)
  Product/1 -> Bus Creator/6  "Charger_pwr_out"
  Bus Selector/4 -> Charger/5(HCU_ChargeHeatingPermission)  "<HCU_ChargeHeatingPermission>"
  Bus Selector/3 -> Charger/4(BMS_MainPosContactorState)  "<BMS_MainPlusContactorCoilState>"

== system HQEV_MiL_20160830_integrate/MiL/Test_Integration/Charger/Charger/Signal ==
  In : Inport
  out : Outport
  wires:
  In/1 -> out/1

== system HQEV_MiL_20160830_integrate/MiL/Test_Integration/Cycle/Cycle/Cycle ==
  In : Inport
  Bus Selector : BusSelector  OutputSignals=Drv.signal2.RunSignal (signal 10)
  SimTimeControl : Subsystem
  Unit Delay : UnitDelay  SampleTime=-1
  velocity_vs_time : Lookup  InputValues=|  Table=|  LookUpMeth=Interpolation-Use End Values  SaturateOnIntegerOverflow=on
      InputValues=|
      | [0
      | 10.23
      | 11
      | 11.77
      | 14.5
      | 15
      | 15.5
      | 22.5
      | 23
      | 23.5
      | 24.5
      | 25
      | 25.5
      | 27.2
      | 28
      | 28.8
      | 48.17
      | 49
      | 49.83
      | 53.5
      | 60.5
      | 61
      | 61.5
      | 84.5
      | 85
      | 85.5
      | 92.5
      | 93
      | 93.5
      | 95.2
      | 96
      | 96.8
      | 116.17
      | 117
      | 117.83
      | 121.5
      | 142.5
      | 143
      | 143.5
      | 154.5
      | 155
      | 155.5
      | 162.5
      | 163
      | 163.5
      | 175.5
      | 176
      | 176.5
      | 177.5
      | 178
      | 178.5
      | 184.5
      | 185
      | 185.5
      | 187.2
      | 188
      | 188.8
      | 194.5
      | 195
      | 195.5
      | 205.23
      | 206
      | 206.77
      | 209.5
      | 210
      | 210.5
      | 217.5
      | 218
      | 218.5
      | 219.5
      | 220
      | 220.5
      | 222.2
      | 223
      | 223.8
      | 243.17
      | 244
      | 244.83
      | 248.5
      | 255.5
      | 256
      | 256.5
      | 279.5
      | 280
      | 280.5
      | 287.5
      | 288
      | 288.5
      | 290.2
      | 291
      | 291.8
      | 311.17
      | 312
      | 312.83
      | 316.5
      | 337.5
      | 338
      | 338.5
      | 349.5
      | 350
      | 350.5
      | 357.5
      | 358
      | 358.5
      | 370.5
      | 371
      | 371.5
      | 372.5
      | 373
      | 373.5
      | 379.5
      | 380
      | 380.5
      | 382.2
      | 383
      | 383.8
      | 389.5
      | 390
      | 390.5
      | 400.23
      | 401
      | 401.77
      | 404.5
      | 405
      | 405.5
      | 412.5
      | 413
      | 413.5
      | 414.5
      | 415
      | 415.5
      | 417.2
      | 418
      | 418.8
      | 438.17
      | 439
      | 439.83
      | 443.5
      | 450.5
      | 451
      | 451.5
      | 474.5
      | 475
      | 475.5
      | 482.5
      | 483
      | 483.5
      | 485.2
      | 486
      | 486.8
      | 506.17
      | 507
      | 507.83
      | 511.5
      | 532.5
      | 533
      | 533.5
      | 544.5
      | 545
      | 545.5
      | 552.5
      | 553
      | 553.5
      | 565.5
      | 566
      | 566.5
      | 567.5
      | 568
      | 568.5
      | 574.5
      | 575
      | 575.5
      | 577.2
      | 578
      | 578.8
      | 584.5
      | 585
      | 585.5
      | 595.23
      | 596
      | 596.77
      | 599.5
      | 600
      | 600.5
      | 607.5
      | 608
      | 608.5
      | 609.5
      | 610
      | 610.5
      | 612.2
      | 613
      | 613.8
      | 633.17
      | 634
      | 634.83
      | 638.5
      | 645.5
      | 646
      | 646.5
      | 669.5
      | 670
      | 670.5
      | 677.5
      | 678
      | 678.5
      | 680.2
      | 681
      | 681.8
      | 701.17
      | 702
      | 702.83
      | 706.5
      | 727.5
      | 728
      | 728.5
      | 739.5
      | 740
      | 740.5
      | 747.5
      | 748
      | 748.5
      | 760.5
      | 761
      | 761.5
      | 762.5
      | 763
      | 763.5
      | 769.5
      | 770
      | 770.5
      | 772.2
      | 773
      | 773.8
      | 779.5
      | 780
      | 780.5
      | 799.17
      | 800
      | 800.83
      | 804.5
      | 840.5
      | 841
      | 841.5
      | 890.5
      | 891
      | 891.5
      | 898.5
      | 899
      | 899.5
      | 967.5
      | 968
      | 968.5
      | 980.5
      | 981
      | 981.5
      | 1030.5
      | 1031
      | 1031.5
      | 1065.5
      | 1066
      | 1066.5
      | 1095.5
      | 1096
      | 1096.5
      | 1115.5
      | 1116
      | 1116.5
      | 1125.5
      | 1126
      | 1126.5
      | 1141.5
      | 1142
      | 1142.5
      | 1149.5
      | 1150
      | 1150.5
      | 1159.3
      | 1160
      | 1160.7
      | 1180
      | ]
      Table=|
      | [0
      | 0
      | 0
      | 2.875
      | 13.125
      | 15
      | 15
      | 15
      | 15
      | 13.75
      | 11.25
      | 10
      | 8.333
      | 2.667
      | 0
      | 0
      | 0
      | 0
      | 2.213
      | 12
      | 30.667
      | 32
      | 32
      | 32
      | 32
      | 30.625
      | 11.375
      | 10
      | 8.333
      | 2.667
      | 0
      | 0
      | 0
      | 0
      | 1.596
      | 8.654
      | 49.038
      | 50
      | 50
      | 50
      | 50
      | 49.062
      | 35.938
      | 35
      | 35
      | 35
      | 35
      | 34.25
      | 32.75
      | 32
      | 30.429
      | 11.571
      | 10
      | 8.333
      | 2.667
      | 0
      | 0
      | 0
      | 0
      | 0
      | 0
      | 0
      | 2.875
      | 13.125
      | 15
      | 15
      | 15
      | 15
      | 13.75
      | 11.25
      | 10
      | 8.333
      | 2.667
      | 0
      | 0
      | 0
      | 0
      | 2.213
      | 12
      | 30.667
      | 32
      | 32
      | 32
      | 32
      | 30.625
      | 11.375
      | 10
      | 8.333
      | 2.667
      | 0
      | 0
      | 0
      | 0
      | 1.596
      | 8.654
      | 49.038
      | 50
      | 50
      | 50
      | 50
      | 49.062
      | 35.938
      | 35
      | 35
      | 35
      | 35
      | 34.25
      | 32.75
      | 32
      | 30.429
      | 11.571
      | 10
      | 8.333
      | 2.667
      | 0
      | 0
      | 0
      | 0
      | 0
      | 0
      | 0
      | 2.875
      | 13.125
      | 15
      | 15
      | 15
      | 15
      | 13.75
      | 11.25
      | 10
      | 8.333
      | 2.667
      | 0
      | 0
      | 0
      | 0
      | 2.213
      | 12
      | 30.667
      | 32
      | 32
      | 32
      | 32
      | 30.625
      | 11.375
      | 10
      | 8.333
      | 2.667
      | 0
      | 0
      | 0
      | 0
      | 1.596
      | 8.654
      | 49.038
      | 50
      | 50
      | 50
      | 50
      | 49.062
      | 35.938
      | 35
      | 35
      | 35
      | 35
      | 34.25
      | 32.75
      | 32
      | 30.429
      | 11.571
      | 10
      | 8.333
      | 2.667
      | 0
      | 0
      | 0
      | 0
      | 0
      | 0
      | 0
      | 2.875
      | 13.125
      | 15
      | 15
      | 15
      | 15
      | 13.75
      | 11.25
      | 10
      | 8.333
      | 2.667
      | 0
      | 0
      | 0
      | 0
      | 2.213
      | 12
      | 30.667
      | 32
      | 32
      | 32
      | 32
      | 30.625
      | 11.375
      | 10
      | 8.333
      | 2.667
      | 0
      | 0
      | 0
      | 0
      | 1.596
      | 8.654
      | 49.038
      | 50
      | 50
      | 50
      | 50
      | 49.062
      | 35.938
      | 35
      | 35
      | 35
      | 35
      | 34.25
      | 32.75
      | 32
      | 30.429
      | 11.571
      | 10
      | 8.333
      | 2.667
      | 0
      | 0
      | 0
      | 0
      | 0
      | 0
      | 0
      | 1.417
      | 7.683
      | 69.146
      | 70
      | 70
      | 70
      | 70
      | 68.75
      | 51.25
      | 50
      | 50
      | 50
      | 50
      | 50.769
      | 69.231
      | 70
      | 70
      | 70
      | 70
      | 70.429
      | 99.571
      | 100
      | 100
      | 100
      | 100
      | 100.5
      | 119.5
      | 120
      | 120
      | 120
      | 120
      | 118.75
      | 81.25
      | 80
      | 78.125
      | 51.875
      | 50
      | 47.5
      | 3.5
      | 0
      | 0
      | 0
      | ]
  v_set [km/h] : Outport  Description=Current set velocity of cycle in [km/h]
  wires:
  SimTimeControl/1(time) -> velocity_vs_time/1
  velocity_vs_time/1 -> v_set [km/h]/1
  In/1 -> Bus Selector/1
  Bus Selector/1 -> Unit Delay/1  "<RunSignal (signal 10)>"
  Unit Delay/1 -> SimTimeControl/1(RunSignal)

== system HQEV_MiL_20160830_integrate/MiL/Test_Integration/DCDC/DCDC/DCDC ==
  In1 : Inport
  Bus Creator : BusCreator  Inputs=7
  Bus Selector : BusSelector  OutputSignals=HCU.HCU_DCDCEnable,HCU.HCU_DCDCOutputVoltageRequest,Battery.Battery_Voltage
  Electric_Manage : Subsystem
  DCDC : Outport
  wires:
  In1/1 -> Electric_Manage/4(IO_In1), Bus Selector/1
  Bus Selector/1 -> Electric_Manage/1(DCDC_enable)  "<HCU_DCDCEnable>"
  Bus Selector/2 -> Electric_Manage/2(V_out_req)  "<HCU_DCDCOutputVoltageRequest>"
  Bus Selector/3 -> Electric_Manage/3(Battery_Voltage)  "<Battery_Voltage>"
  Electric_Manage/1(DCDC_Status) -> Bus Creator/1  "DCDC_Status"
  Electric_Manage/2(DCDC_pwr_Output) -> Bus Creator/2  "DCDC_Output_Power"
  Electric_Manage/3(DCDC_pwr_Input) -> Bus Creator/3  "DCDC_Input_Power"
  Electric_Manage/4(DCDC_I_Input) -> Bus Creator/4  "DCDC_Input_Current"
  Electric_Manage/5(DCDC_U_Input) -> Bus Creator/5  "DCDC_Input_Voltage"
  Electric_Manage/6(DCDC_I_Output) -> Bus Creator/6  "DCDC_Output_Current"
  Electric_Manage/7(DCDC_U_Output) -> Bus Creator/7  "DCDC_Output_Voltage"
  Bus Creator/1 -> DCDC/1

== system HQEV_MiL_20160830_integrate/MiL/Test_Integration/DCDC/DCDC/Output ==
  In1 : Inport
  Bus Creator : BusCreator  Inputs=10
  Checksum_DCDC1 : Subsystem
  DCDCLoss : Subsystem
  DCDC_InputCurrent : Subsystem
  DCDC_InputVoltage : Subsystem
  DCDC_Input_Powr : Subsystem
  DCDC_OutputCurrent : Subsystem
  DCDC_OutputVoltage : Subsystem
  DCDC_Status : Subsystem
  DCDC_Temperature : Subsystem
  LiveCounter_DCDC_1 : Subsystem
  Out1 : Outport
  wires:
  Checksum_DCDC1/1(Checksum_DCDC1) -> Bus Creator/1  "Checksum_DCDC1"
  DCDC_OutputCurrent/1(DCDC_Output_Current) -> Bus Creator/2  "DCDC_OutputCurrent"
  DCDC_Status/1(DCDC_Status) -> Bus Creator/3  "DCDC_Status"
  LiveCounter_DCDC_1/1(LiveCounter_DCDC1) -> Bus Creator/4  "LiveCounter_DCDC_1"
  DCDC_OutputVoltage/1(DCDC_Output_Voltage) -> Bus Creator/5  "DCDC_OutputVoltage"
  DCDC_InputCurrent/1(DCDC_in_Current) -> Bus Creator/6  "DCDC_InputCurrent"
  DCDC_Temperature/1(DCDC_Temperature) -> Bus Creator/8  "DCDC_Temperature"
  DCDC_InputVoltage/1(DCDC_Input_Voltage) -> Bus Creator/9  "DCDC_InputVoltage"
  In1/1 -> Checksum_DCDC1/1(In1), DCDC_OutputCurrent/1(In), DCDC_Status/1(In1), LiveCounter_DCDC_1/1(In1), DCDCLoss/1(In1), DCDC_InputVoltage/1(In1), DCDC_Input_Powr/1(In1), DCDC_InputCurrent/1(In1), DCDC_OutputVoltage/1(In1)
  DCDC_Input_Powr/1(DCDC_Input_Power) -> Bus Creator/7  "DCDC_Input_Powr"
  DCDCLoss/1(pwr_DCDCLoss) -> Bus Creator/10  "DCDC_pwr_Loss"
  Bus Creator/1 -> Out1/1

== system HQEV_MiL_20160830_integrate/MiL/Test_Integration/Driver/Driver/Control_Panel ==
  IO_IN : Inport
  ACButton : Subsystem
  ACC_Cruise_Button : Subsystem
  ACStation_U : Subsystem
  Bus Creator : BusCreator  Inputs=16
  CP : Subsystem
  EGSM_ECOSButton : Subsystem
  EGSM_KnobPosition : Subsystem
  EGSM_ParkButton : Subsystem
  EGSM_SecurityButton : Subsystem
  FastCharge : Subsystem
  InterlockA : Subsystem
  InterlockB : Subsystem
  KeyONState : Subsystem
  KeyStartState : Subsystem
  LeverPosition : Subsystem
  RunSignal : Subsystem
  Out1 : Outport
  wires:
  Bus Creator/1 -> Out1/1
  IO_IN/1 -> InterlockB/1(IO_IN), ACC_Cruise_Button/1(IO_IN), ACButton/1(IO_IN), FastCharge/1(IO_IN), KeyStartState/1(IO_IN), KeyONState/1(IO_IN), InterlockA/1(IO_IN), LeverPosition/1(IO_IN)
  LeverPosition/1(out) -> Bus Creator/1  "Lever_Position"
  InterlockA/1(out) -> Bus Creator/2  "interlockA"
  InterlockB/1(out) -> Bus Creator/3  "InterlockB"
  KeyONState/1(out) -> Bus Creator/4  "KeyONState"
  KeyStartState/1(out) -> Bus Creator/5  "KeyStartState"
  FastCharge/1(out) -> Bus Creator/7, Bus Creator/6  "FastCharge"
  CP/1(out) -> Bus Creator/8  "CP"
  ACStation_U/1(out) -> Bus Creator/9  "ACStation_U"
  RunSignal/1(out) -> Bus Creator/10  "RunSignal"
  EGSM_ParkButton/1(out) -> Bus Creator/11  "ParkButton"
  EGSM_SecurityButton/1(out) -> Bus Creator/12  "SecurityButton"
  EGSM_KnobPosition/1(out) -> Bus Creator/13  "EGSM_KnobPosition"
  EGSM_ECOSButton/1(out) -> Bus Creator/14  "EGSM_ECOSButton"
  ACButton/1(out) -> Bus Creator/15  "ACButton"
  ACC_Cruise_Button/1(out) -> Bus Creator/16  "ACC_CruiseButton"

== system HQEV_MiL_20160830_integrate/MiL/Test_Integration/Driver/Driver/Driver_AutoPedal ==
  Veh_v : Inport
  Cycle_v_set : Inport  Port=2
  Bus Creator : BusCreator  Inputs=2
  Bus Creator1 : BusCreator  Inputs=2
  Bus Creator2 : BusCreator  Inputs=3
  Bus Selector : BusSelector  OutputSignals=Sig_AccPed_pct,Sig_BrkPed_pct
  Bus Selector1 : BusSelector  OutputSignals=v_Set
  Bus Selector2 : BusSelector  OutputSignals=v_Set,v_Veh,Brake
  Bus Selector3 : BusSelector  OutputSignals=v_Set,v_Veh
  CTRL AccPed : Subsystem
  CTRL BrakePed : Subsystem
  Compare To Constant : simulink/Logic and Bit Operations/Compare To Constant  SystemSampleTime=-1  relop=>  const=1  LogicOutDataTypeMode=uint8
  Constant1 : Constant  Value=100
  Constant3 : Constant  Value=0
  Data Type Conversion : DataTypeConversion
  Stop_Indicator : Subsystem
  Switch2 : Switch  Criteria=u2 > Threshold
  Unit Delay : UnitDelay  SampleTime=-1
  Unit Delay1 : UnitDelay  SampleTime=-1
  AccPed_pct : Outport
  BrkPed_pct : Outport  Port=2
  Brake_OnOff : Outport  Port=3
  wires:
  CTRL AccPed/1(Sig_AccPed [%]) -> Bus Creator1/1  "Sig_AccPed_pct"
  Constant3/1 -> Bus Creator/1  "Sig_AccPed_pct"
  Constant1/1 -> Bus Creator/2  "Sig_BrkPed_pct"
  Bus Creator/1 -> Switch2/1
  Bus Creator1/1 -> Switch2/3
  Switch2/1 -> Bus Selector/1
  Stop_Indicator/1(stop) -> Switch2/2
  Bus Selector/1 -> Unit Delay1/1  "<Sig_AccPed_pct>"
  Bus Selector/2 -> Unit Delay/1  "<Sig_BrkPed_pct>"
  CTRL BrakePed/1("Brake[%] ") -> Bus Creator1/2  "Sig_BrkPed_pct"
  Veh_v/1 -> Bus Creator2/1
  Cycle_v_set/1 -> Bus Creator2/2
  Bus Creator2/1 -> Bus Selector1/1, Bus Selector2/1, Bus Selector3/1
  Bus Selector1/1 -> Stop_Indicator/1(v_set)  "<v_Set>"
  Bus Selector2/1 -> CTRL AccPed/1(v_set [km/h])  "<v_Set>"
  Bus Selector2/2 -> CTRL AccPed/2(v_Veh [km/h])  "<v_Veh>"
  Bus Selector2/3 -> CTRL AccPed/3(Brake [%])  "<Brake>"
  Bus Selector3/1 -> CTRL BrakePed/1(v_set [km/h])  "<v_Set>"
  Bus Selector3/2 -> CTRL BrakePed/2(v_Veh [km/h])  "<v_Veh>"
  Unit Delay/1 -> BrkPed_pct/1, Bus Creator2/3, Compare To Constant/1  "Brake"
  Compare To Constant/1 -> Data Type Conversion/1
  Data Type Conversion/1 -> Brake_OnOff/1
  Unit Delay1/1 -> AccPed_pct/1

== system HQEV_MiL_20160830_integrate/MiL/Test_Integration/Driver/Driver/Driver_ManualPedal ==
  IO_IN : Inport
  Bus Selector : BusSelector  OutputSignals=AccPed,BrakePed
  Compare To Constant : simulink/Logic and Bit Operations/Compare To Constant  SystemSampleTime=-1  relop=>  const=1  LogicOutDataTypeMode=uint8
  Data Type Conversion : DataTypeConversion
  AccPed_pct : Outport
  BrkPed_pct : Outport  Port=2
  Brake_OnOff : Outport  Port=3
  wires:
  Bus Selector/2 -> Compare To Constant/1, BrkPed_pct/1  "<BrakePed>"
  Compare To Constant/1 -> Data Type Conversion/1
  Data Type Conversion/1 -> Brake_OnOff/1
  Bus Selector/1 -> AccPed_pct/1  "<AccPed>"
  IO_IN/1 -> Bus Selector/1

== system HQEV_MiL_20160830_integrate/MiL/Test_Integration/EBS/EBS/Subsystem ==
  Constant : Constant  Value=90
  SOC : Outport
  wires:
  Constant/1 -> SOC/1

== system HQEV_MiL_20160830_integrate/MiL/Test_Integration/EBS/EBS/Subsystem1 ==
  Constant1 : Constant  Value=25
  T_BATT : Outport
  wires:
  Constant1/1 -> T_BATT/1

== system HQEV_MiL_20160830_integrate/MiL/Test_Integration/EBS/EBS/Subsystem2 ==
  Constant2 : Constant  Value=0
  Status_Temp : Outport
  wires:
  Constant2/1 -> Status_Temp/1

== system HQEV_MiL_20160830_integrate/MiL/Test_Integration/EBS/EBS/Subsystem3 ==
  Constant3 : Constant  Value=0
  ERROR_Calib : Outport
  wires:
  Constant3/1 -> ERROR_Calib/1

== system HQEV_MiL_20160830_integrate/MiL/Test_Integration/EBS/EBS/Subsystem4 ==
  Constant4 : Constant  Value=0
  Resp_Error : Outport
  wires:
  Constant4/1 -> Resp_Error/1

== system HQEV_MiL_20160830_integrate/MiL/Test_Integration/EBS/EBS/Subsystem5 ==
  Constant5 : Constant  Value=0
  FLAG_INCONSISTENCY : Outport
  wires:
  Constant5/1 -> FLAG_INCONSISTENCY/1

== system HQEV_MiL_20160830_integrate/MiL/Test_Integration/EBS/EBS/Subsystem6 ==
  Constant6 : Constant
  SOC_STATE : Outport
  wires:
  Constant6/1 -> SOC_STATE/1

== system HQEV_MiL_20160830_integrate/MiL/Test_Integration/EBS/EBS/Subsystem7 ==
  Constant : Constant  Value=90
  out : Outport
  wires:
  Constant/1 -> out/1

== system HQEV_MiL_20160830_integrate/MiL/Test_Integration/EPS/EPS/Subsystem2 ==
  Subsystem : Subsystem
  Subsystem1 : Subsystem
  EPSErrorStatus : Outport
  SteeringWheelAngleStatus : Outport  Port=2
  wires:
  Subsystem/1(EPSErrorStatus) -> EPSErrorStatus/1
  Subsystem1/1(SteeringWheelAngleStatus) -> SteeringWheelAngleStatus/1
